simulink model "directRRR"  (R2021b)
settings: Solver=VariableStepAuto  StartTime=0.0  StopTime=10.0  RelTol=1e-3
settings Model: Creator=fabioscap  LastModifiedBy=fabioscap

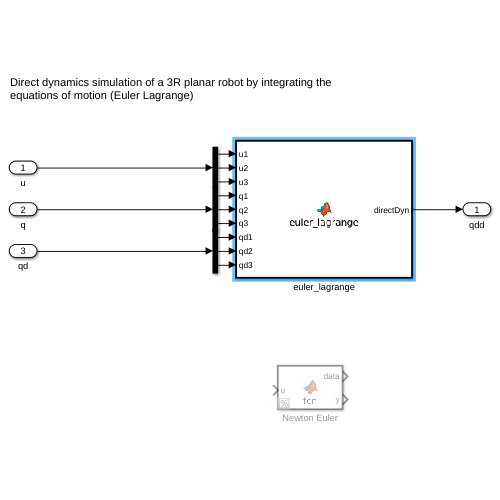
[thumbnail: Simulink's stored preview of the top-level diagram]
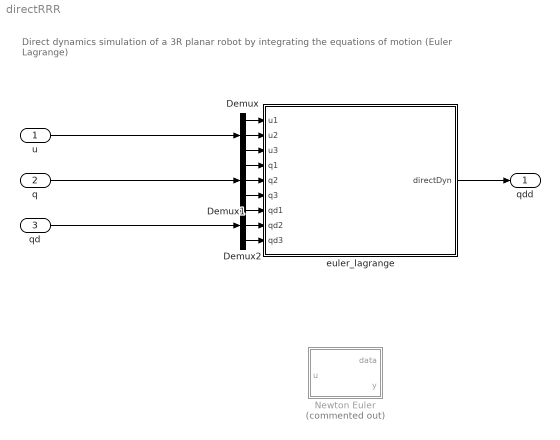
== system directRRR ==
  note: Direct dynamics simulation of a 3R planar robot by integrating the equations of motion (Euler Lagrange)
  u : Inport  PortDimensions=3
  q : Inport  Port=2  PortDimensions=3
  qd : Inport  Port=3  PortDimensions=3
  Demux : Demux  Outputs=3
  Demux1 : Demux  Outputs=3
  Demux2 : Demux  Outputs=3
  Newton Euler : MATLAB Function  Commented=on  TreatAsAtomicUnit=on
  euler_lagrange : MATLAB Function  TreatAsAtomicUnit=on
  qdd : Outport  PortDimensions=3
  wires:
  u/1 -> Demux/1
  Demux2/1 -> euler_lagrange/7(qd1)
  Demux2/3 -> euler_lagrange/9(qd3)
  Demux1/1 -> euler_lagrange/4(q1)
  Demux1/2 -> euler_lagrange/5(q2)
  Demux1/3 -> euler_lagrange/6(q3)
  Demux/3 -> euler_lagrange/3(u3)
  Demux/2 -> euler_lagrange/2(u2)
  Demux/1 -> euler_lagrange/1(u1)
  Demux2/2 -> euler_lagrange/8(qd2)
  euler_lagrange/1(directDyn) -> qdd/1
  qd/1 -> Demux2/1
  q/1 -> Demux1/1

== matlab function directRRR/euler_lagrange ==
  data: u1 input; directDyn output; u2 input; u3 input; q1 input; q2 input; q3 input; qd1 input; qd2 input; qd3 input
function directDyn = euler_lagrange(u1,u2,u3,q1,q2,q3,qd1,qd2,qd3)
%#codegen

%    This function was generated by the Symbolic Math Toolbox version 9.0.
%    20-Jul-2022 19:34:33

t2 = cos(q1);
t3 = cos(q2);
t4 = cos(q3);
t5 = sin(q1);
t6 = sin(q2);
t7 = sin(q3);
t8 = q2+q3;
t9 = qd1.^2;
t10 = qd2.^2;
t11 = qd3.^2;
t23 = u1.*5.0e+3;
t12 = t3.^2;
t13 = t3.^3;
t14 = t4.^2;
t15 = t4.^3;
t16 = t7.^2;
t17 = t7.^3;
t18 = cos(t8);
t19 = sin(t8);
t28 = t3.*u1.*2.0e+3;
t29 = t3.*u2.*2.0e+3;
t30 = t3.*u3.*2.0e+3;
t31 = t2.*1.22625e+5;
t35 = t7.*t11.*4.5e+3;
t36 = t6.*t10.*7.5e+3;
t39 = qd1.*qd3.*t7.*9.0e+3;
t40 = qd2.*qd3.*t7.*9.0e+3;
t41 = qd1.*qd2.*t6.*1.5e+4;
t46 = t3.*t4.*u3.*8.0e+2;
t48 = t2.*t3.*8.3385e+4;
t53 = t5.*t6.*1.32435e+5;
t58 = qd1.*qd2.*t3.*t7.*2.0e+3;
t59 = qd1.*qd3.*t3.*t7.*2.0e+3;
t60 = qd2.*qd3.*t3.*t7.*2.0e+3;
t61 = qd1.*qd2.*t3.*t6.*6.0e+3;
t77 = t3.*t7.*t9.*1.0e+3;
t78 = t3.*t7.*t10.*1.0e+3;
t79 = t3.*t7.*t11.*1.0e+3;
t80 = t3.*t6.*t9.*3.0e+3;
t81 = t3.*t6.*t10.*3.0e+3;
t85 = t3.*t5.*t6.*2.943e+4;
t91 = t3.*t4.*t7.*t9.*4.0e+2;
t92 = t3.*t4.*t7.*t10.*4.0e+2;
t98 = qd1.*qd2.*t3.*t4.*t7.*8.0e+2;
t128 = t2.*t4.*t6.*t7.*1.7658e+4;
t129 = t3.*t4.*t5.*t7.*1.7658e+4;
t144 = t2.*t3.*t4.*t6.*t7.*3.924e+3;
t20 = t18.^2;
t21 = t19.^2;
t22 = t19.^3;
t24 = t12.*2.0e+1;
t26 = t14.*1.44e+2;
t27 = t16.*1.8e+2;
t32 = -t29;
t33 = t14.*u1.*3.2e+3;
t34 = t14.*u2.*3.2e+3;
t37 = t16.*u1.*4.0e+3;
t38 = t16.*u2.*4.0e+3;
t42 = -t31;
t45 = t18.*u3.*2.0e+3;
t49 = -t35;
t51 = -t39;
t52 = -t40;
t55 = qd1.*qd2.*t19.*5.0e+3;
t56 = qd1.*qd3.*t19.*5.0e+3;
t57 = qd2.*qd3.*t19.*5.0e+3;
t62 = -t53;
t63 = t4.*t18.*u1.*3.2e+3;
t64 = t4.*t18.*u2.*3.2e+3;
t65 = t4.*t18.*u3.*3.2e+3;
t66 = t2.*t12.*2.943e+4;
t67 = t7.*t19.*u1.*4.0e+3;
t68 = t7.*t19.*u2.*4.0e+3;
t69 = t7.*t19.*u3.*4.0e+3;
t70 = t3.*t4.*t18.*6.4e+1;
t71 = t3.*t7.*t19.*8.0e+1;
t73 = t9.*t19.*2.5e+3;
t74 = t10.*t19.*2.5e+3;
t75 = t11.*t19.*2.5e+3;
t82 = -t58;
t83 = -t59;
t84 = -t60;
t87 = t2.*t14.*7.848e+4;
t89 = t2.*t16.*9.81e+4;
t93 = qd1.*qd2.*t3.*t19.*2.0e+3;
t94 = qd1.*qd2.*t7.*t18.*2.0e+3;
t95 = qd1.*qd3.*t3.*t19.*2.0e+3;
t96 = qd2.*qd3.*t3.*t19.*2.0e+3;
t101 = -t77;
t102 = -t78;
t103 = -t79;
t104 = -t85;
t105 = t2.*t3.*t14.*1.7658e+4;
t106 = t4.*t7.*t19.*u3.*1.6e+3;
t107 = t6.*t9.*t14.*4.8e+3;
t108 = t6.*t10.*t14.*4.8e+3;
t109 = t6.*t9.*t16.*6.0e+3;
t110 = t6.*t10.*t16.*6.0e+3;
t111 = qd1.*qd2.*t6.*t14.*9.6e+3;
t112 = t5.*t6.*t14.*1.7658e+4;
t114 = qd1.*qd2.*t6.*t16.*1.2e+4;
t118 = t3.*t9.*t19.*1.0e+3;
t119 = t7.*t9.*t18.*1.0e+3;
t120 = t3.*t10.*t19.*1.0e+3;
t121 = t7.*t10.*t18.*1.0e+3;
t122 = t3.*t11.*t19.*1.0e+3;
t123 = t4.*t9.*t19.*1.8e+3;
t124 = t16.*t18.*u3.*1.6e+3;
t125 = -t91;
t126 = -t92;
t127 = -t98;
t130 = qd1.*qd2.*t17.*t18.*1.6e+3;
t131 = qd1.*qd2.*t14.*t19.*3.2e+3;
t132 = qd1.*qd3.*t14.*t19.*3.2e+3;
t134 = qd2.*qd3.*t14.*t19.*3.2e+3;
t136 = t3.*t5.*t6.*t14.*3.924e+3;
t137 = t4.*t5.*t7.*t12.*3.924e+3;
t139 = t3.*t4.*t9.*t19.*4.0e+2;
t140 = t2.*t12.*t14.*3.924e+3;
t141 = qd1.*qd2.*t4.*t7.*t18.*3.2e+3;
t142 = qd1.*qd3.*t4.*t7.*t18.*3.2e+3;
t143 = qd2.*qd3.*t4.*t7.*t18.*3.2e+3;
t145 = t2.*t4.*t18.*7.848e+4;
t148 = t2.*t7.*t19.*9.81e+4;
t150 = t9.*t17.*t18.*8.0e+2;
t152 = t10.*t17.*t18.*8.0e+2;
t153 = t9.*t14.*t19.*1.6e+3;
t154 = t10.*t14.*t19.*1.6e+3;
t155 = t11.*t14.*t19.*1.6e+3;
t164 = t4.*t7.*t18.*t19.*1.28e+2;
t165 = t2.*t3.*t4.*t18.*5.6898e+4;
t166 = t9.*t18.*t19.*1.0e+3;
t168 = t4.*t7.*t9.*t18.*1.6e+3;
t169 = t4.*t7.*t10.*t18.*1.6e+3;
t170 = t4.*t7.*t11.*t18.*1.6e+3;
t171 = t4.*t6.*t9.*t18.*4.8e+3;
t172 = t4.*t6.*t10.*t18.*4.8e+3;
t177 = qd1.*qd2.*t4.*t6.*t18.*9.6e+3;
t178 = t2.*t6.*t7.*t18.*9.81e+3;
t179 = t3.*t5.*t7.*t18.*9.81e+3;
t180 = t4.*t5.*t6.*t18.*5.6898e+4;
t181 = t2.*t3.*t7.*t19.*5.886e+4;
t183 = t6.*t7.*t9.*t19.*6.0e+3;
t184 = t6.*t7.*t10.*t19.*6.0e+3;
t185 = qd1.*qd2.*t6.*t7.*t19.*1.2e+4;
t186 = t5.*t6.*t7.*t19.*5.886e+4;
t188 = t5.*t7.*t12.*t18.*3.924e+3;
t189 = t2.*t6.*t17.*t18.*7.848e+3;
t190 = t3.*t5.*t17.*t18.*7.848e+3;
t191 = qd1.*qd2.*t4.*t16.*t19.*1.6e+3;
t197 = t3.*t9.*t18.*t19.*4.0e+2;
t198 = qd1.*qd2.*t4.*t18.*t19.*3.2e+3;
t199 = qd1.*qd3.*t4.*t18.*t19.*3.2e+3;
t200 = qd2.*qd3.*t4.*t18.*t19.*3.2e+3;
t202 = t2.*t3.*t6.*t7.*t18.*3.924e+3;
t203 = t3.*t4.*t5.*t6.*t18.*3.924e+3;
t211 = t2.*t4.*t12.*t18.*3.924e+3;
t217 = t4.*t9.*t18.*t19.*1.6e+3;
t218 = t4.*t10.*t18.*t19.*1.6e+3;
t219 = t4.*t11.*t18.*t19.*1.6e+3;
t222 = t4.*t9.*t16.*t19.*8.0e+2;
t224 = t4.*t10.*t16.*t19.*8.0e+2;
t228 = t2.*t3.*t4.*t16.*t18.*7.848e+3;
t229 = t2.*t3.*t7.*t14.*t19.*7.848e+3;
t230 = qd1.*qd2.*t16.*t18.*t19.*1.6e+3;
t231 = t4.*t5.*t6.*t16.*t18.*7.848e+3;
t232 = t2.*t4.*t6.*t16.*t19.*7.848e+3;
t233 = t3.*t4.*t5.*t16.*t19.*7.848e+3;
t236 = t5.*t6.*t7.*t14.*t19.*7.848e+3;
t242 = t9.*t16.*t18.*t19.*8.0e+2;
t244 = t10.*t16.*t18.*t19.*8.0e+2;
t247 = t2.*t3.*t4.*t7.*t18.*t19.*7.848e+3;
t248 = t4.*t5.*t6.*t7.*t18.*t19.*7.848e+3;
t249 = t2.*t6.*t16.*t18.*t19.*7.848e+3;
t250 = t3.*t5.*t16.*t18.*t19.*7.848e+3;
t25 = -t24;
t43 = t20.*8.0e+1;
t44 = t21.*1.0e+2;
t47 = -t34;
t50 = -t38;
t54 = -t45;
t72 = t20.*u2.*3.2e+3;
t76 = t21.*u2.*4.0e+3;
t86 = -t64;
t88 = -t68;
t90 = -t70;
t97 = -t71;
t113 = -t87;
t115 = -t89;
t116 = t16.*t20.*6.4e+1;
t117 = t14.*t21.*6.4e+1;
t133 = qd1.*qd3.*t7.*t20.*3.2e+3;
t135 = qd2.*qd3.*t7.*t20.*3.2e+3;
t138 = -t105;
t146 = -t123;
t147 = -t124;
t149 = t2.*t3.*t20.*4.7088e+4;
t151 = t4.*t9.*t22.*8.0e+2;
t156 = t7.*t11.*t20.*1.6e+3;
t157 = t6.*t9.*t20.*4.8e+3;
t158 = t2.*t3.*t21.*5.886e+4;
t159 = t6.*t9.*t21.*6.0e+3;
t162 = t5.*t6.*t20.*4.7088e+4;
t163 = t5.*t6.*t21.*5.886e+4;
t167 = -t139;
t173 = -t140;
t174 = -t141;
t175 = -t142;
t176 = -t143;
t182 = -t145;
t187 = -t148;
t192 = qd1.*qd2.*t4.*t7.*t21.*1.6e+3;
t201 = -t164;
t204 = -t168;
t205 = -t169;
t206 = -t170;
t207 = -t178;
t208 = -t179;
t209 = -t180;
t210 = -t186;
t212 = -t188;
t213 = -t189;
t214 = -t190;
t215 = -t191;
t220 = -t202;
t221 = -t203;
t223 = t4.*t7.*t9.*t21.*8.0e+2;
t225 = t4.*t7.*t10.*t21.*8.0e+2;
t226 = t2.*t3.*t14.*t21.*7.848e+3;
t227 = t5.*t6.*t14.*t21.*7.848e+3;
t234 = t2.*t4.*t6.*t7.*t21.*7.848e+3;
t235 = t3.*t4.*t5.*t7.*t21.*7.848e+3;
t237 = -t222;
t239 = -t224;
t243 = t7.*t9.*t18.*t21.*8.0e+2;
t245 = -t229;
t246 = -t231;
t251 = -t248;
t252 = -t249;
t253 = -t250;
t99 = -t72;
t100 = -t76;
t160 = -t133;
t161 = -t135;
t193 = -t151;
t194 = -t156;
t195 = -t162;
t196 = -t163;
t216 = -t192;
t238 = -t223;
t240 = -t225;
t241 = -t226;
t254 = t25+t26+t27+t43+t44+t90+t97+t116+t117+t201+2.25e+2;
t255 = 1.0./t254;
et1 = t23+t28+t30+t33+t36+t37+t41+t42+t46+t47+t48+t49+t50+t51+t52+t54+t55+t56+t57+t61+t62+t63+t65+t66+t67+t69+t73+t74+t75+t81+t82+t83+t84+t93+t94+t95+t96+t99+t100+t101+t102+t103+t104+t106+t107+t108+t109+t110+t111+t112+t113+t114+t115+t118+t119+t120+t121+t122+t125+t126+t127+t128+t129+t130+t131+t132+t134+t136+t137+t138+t144+t146+t147+t149+t150+t152+t153+t154+t155+t157+t158+t159+t160+t161+t165+t166+t167+t172+t173+t174+t175+t176+t177+t181+t182+t184+t185+t187+t193+t194+t195+t196+t197+t198+t199+t200+t204+t205+t206+t207+t208+t209+t210+t211+t212+t213+t214+t215+t216+t217+t218+t219+t220+t221+t227+t228+t230+t232+t233+t234+t235+t236+t237+t239+t240+t241+t243+t244+t245+t246+t247+t251+t252+t253-u2.*1.4e+4+u3.*9.0e+3+t6.*t9.*2.1e+4-t7.*t9.*4.5e+3-t7.*t10.*4.5e+3-t3.*u2.*4.0e+3+t4.*u3.*3.6e+3;
et2 = t20.*u3.*3.2e+3+t21.*u3.*4.0e+3-qd1.*qd2.*t7.*9.0e+3+t3.*t6.*t9.*6.0e+3-t4.*t7.*t9.*1.8e+3-t4.*t7.*t10.*1.8e+3-t7.*t9.*t20.*1.6e+3-t7.*t10.*t20.*1.6e+3-t3.*t18.*u3.*8.0e+2-t4.*t18.*u2.*6.4e+3+t4.*t21.*u3.*1.6e+3-t7.*t19.*u2.*8.0e+3-qd1.*qd2.*t4.*t7.*3.6e+3-qd1.*qd2.*t7.*t20.*3.2e+3+t3.*t7.*t9.*t18.*4.0e+2+t4.*t6.*t9.*t18.*9.6e+3+t3.*t7.*t10.*t18.*4.0e+2-t4.*t7.*t9.*t21.*1.6e+3+t6.*t7.*t9.*t19.*1.2e+4+t9.*t16.*t18.*t19.*1.6e+3-t7.*t18.*t19.*u3.*1.6e+3+qd1.*qd2.*t3.*t7.*t18.*8.0e+2;
et3 = t28+t32+t48+t49+t51+t52+t61+t62+t63+t67+t80+t81+t86+t88+t93+t95+t96+t99+t100+t112+t118+t120+t122+t128+t129+t138+t139+t146+t149+t157+t158+t159+t160+t161-t166+t171+t172+t177+t182+t183+t184+t185+t187+t193+t194+t195+t196+t197+t198+t199+t200+t211+t212+t216+t217+t218+t219+t220+t221+t227+t230+t234+t235+t238+t240+t241+t242+t243+t244+t247+t251+t252+t253-u2.*9.0e+3+u3.*1.8e+4+t6.*t9.*1.35e+4-t7.*t9.*9.0e+3-t7.*t10.*9.0e+3+t2.*t18.*4.905e+4-t9.*t17.*3.6e+3-t10.*t17.*3.6e+3-t9.*t19.*4.5e+3-t9.*t22.*2.0e+3+t3.*t141+t3.*t168+t3.*t169+t3.*t217-t4.*u2.*3.6e+3+t4.*u3.*7.2e+3-t12.*u3.*8.0e+2+t14.*u3.*7.2e+3;
et4 = t16.*u3.*7.2e+3-t18.*u1.*2.0e+3+t18.*u2.*2.0e+3+t20.*u3.*7.2e+3+t21.*u3.*8.0e+3-qd1.*qd2.*t7.*1.8e+4-qd1.*qd2.*t17.*7.2e+3-t2.*t3.*t4.*1.0791e+4+t2.*t6.*t7.*4.4145e+4+t3.*t5.*t7.*4.4145e+4-t4.*t5.*t6.*8.829e+3+t2.*t4.*t13.*3.924e+3+t4.*t6.*t9.*5.4e+3-t2.*t3.*t15.*3.5316e+4-t4.*t7.*t9.*3.6e+3-t4.*t7.*t10.*3.6e+3-t4.*t7.*t11.*1.8e+3+t2.*t6.*t17.*3.5316e+4+t3.*t5.*t17.*3.5316e+4-t5.*t7.*t13.*3.924e+3+t5.*t6.*t15.*3.5316e+4+t7.*t9.*t12.*4.0e+2+t7.*t10.*t12.*4.0e+2;
et5 = t7.*t9.*t14.*-3.6e+3-t7.*t10.*t14.*3.6e+3-t2.*t12.*t18.*1.1772e+4-t6.*t9.*t18.*3.0e+3-t6.*t10.*t18.*3.0e+3+t2.*t16.*t18.*3.924e+4-t7.*t9.*t20.*3.6e+3-t7.*t9.*t21.*2.0e+3-t7.*t10.*t20.*3.6e+3-t7.*t10.*t21.*2.0e+3+t9.*t12.*t19.*4.0e+2-t9.*t14.*t19.*3.6e+3-t9.*t16.*t19.*3.6e+3-t9.*t14.*t22.*1.6e+3-t9.*t17.*t20.*1.6e+3-t10.*t17.*t20.*1.6e+3-t10.*t18.*t19.*1.0e+3-t9.*t19.*t20.*2.0e+3-t11.*t18.*t19.*1.0e+3+t3.*t4.*u1.*8.0e+2-t3.*t4.*u2.*8.0e+2+t3.*t18.*u2.*8.0e+2;
et6 = t3.*t18.*u3.*-1.6e+3-t4.*t21.*u2.*1.6e+3+t4.*t21.*u3.*3.2e+3-t16.*t18.*u1.*1.6e+3+t16.*t18.*u2.*1.6e+3+t14.*t21.*u3.*3.2e+3+t16.*t20.*u3.*3.2e+3-qd1.*qd2.*t4.*t7.*7.2e+3-qd1.*qd3.*t4.*t7.*3.6e+3-qd2.*qd3.*t4.*t7.*3.6e+3+qd1.*qd2.*t7.*t12.*8.0e+2-qd1.*qd2.*t7.*t14.*7.2e+3-qd1.*qd2.*t6.*t18.*6.0e+3-qd1.*qd2.*t7.*t20.*7.2e+3-qd1.*qd2.*t7.*t21.*4.0e+3-qd1.*qd2.*t17.*t20.*3.2e+3-qd1.*qd2.*t18.*t19.*2.0e+3-qd1.*qd3.*t18.*t19.*2.0e+3-qd2.*qd3.*t18.*t19.*2.0e+3+t3.*t4.*t6.*t9.*1.2e+3+t3.*t4.*t6.*t10.*1.2e+3;
et7 = t2.*t3.*t4.*t16.*-3.5316e+4-t2.*t6.*t7.*t12.*3.924e+3-t4.*t5.*t6.*t12.*3.924e+3-t2.*t3.*t4.*t20.*1.962e+4+t2.*t6.*t7.*t14.*3.5316e+4+t3.*t5.*t7.*t14.*3.5316e+4+t2.*t3.*t4.*t21.*3.924e+3+t4.*t5.*t6.*t16.*3.5316e+4-t2.*t4.*t7.*t19.*3.924e+4+t3.*t5.*t6.*t18.*1.1772e+4+t2.*t6.*t7.*t20.*1.962e+4+t3.*t5.*t7.*t20.*1.962e+4+t4.*t5.*t6.*t20.*1.962e+4+t2.*t6.*t7.*t21.*1.962e+4+t3.*t4.*t10.*t19.*4.0e+2+t3.*t5.*t7.*t21.*1.962e+4-t3.*t6.*t9.*t18.*1.2e+3-t4.*t5.*t6.*t21.*3.924e+3+t3.*t4.*t11.*t19.*4.0e+2+t3.*t7.*t9.*t18.*8.0e+2;
et8 = t3.*t7.*t10.*t18.*8.0e+2+t3.*t7.*t11.*t18.*4.0e+2+t3.*t7.*t9.*t21.*1.6e+3+t4.*t6.*t9.*t21.*2.4e+3-t2.*t3.*t15.*t21.*1.5696e+4+t2.*t6.*t17.*t20.*1.5696e+4+t3.*t5.*t17.*t20.*1.5696e+4+t2.*t12.*t14.*t18.*1.5696e+4+t3.*t9.*t16.*t19.*1.6e+3+t5.*t6.*t15.*t21.*1.5696e+4+t3.*t10.*t16.*t19.*1.6e+3-t6.*t9.*t16.*t18.*2.4e+3-t6.*t10.*t16.*t18.*2.4e+3-t7.*t9.*t14.*t21.*1.6e+3-t5.*t12.*t16.*t19.*1.5696e+4-t7.*t10.*t14.*t21.*1.6e+3-t9.*t16.*t19.*t20.*1.6e+3-t3.*t4.*t18.*u3.*3.2e+3+t4.*t7.*t19.*u1.*1.6e+3-t3.*t7.*t19.*u3.*3.2e+3;
et9 = t4.*t7.*t19.*u2.*-1.6e+3+t7.*t18.*t19.*u2.*1.6e+3-t7.*t18.*t19.*u3.*3.2e+3+qd1.*qd2.*t3.*t4.*t6.*2.4e+3+qd1.*qd2.*t3.*t4.*t19.*8.0e+2+qd1.*qd3.*t3.*t4.*t19.*8.0e+2+qd1.*qd2.*t3.*t7.*t18.*1.6e+3+qd2.*qd3.*t3.*t4.*t19.*8.0e+2+qd1.*qd3.*t3.*t7.*t18.*8.0e+2+qd2.*qd3.*t3.*t7.*t18.*8.0e+2+qd1.*qd2.*t3.*t16.*t19.*3.2e+3-qd1.*qd2.*t6.*t16.*t18.*4.8e+3-qd1.*qd2.*t7.*t14.*t21.*3.2e+3+t2.*t4.*t7.*t12.*t19.*1.5696e+4-t2.*t3.*t4.*t16.*t20.*1.5696e+4+t4.*t6.*t7.*t9.*t19.*2.4e+3-t2.*t3.*t6.*t16.*t19.*1.5696e+4-t3.*t5.*t6.*t14.*t18.*1.5696e+4-t4.*t5.*t7.*t12.*t18.*1.5696e+4;
et10 = t4.*t6.*t7.*t10.*t19.*2.4e+3-t2.*t3.*t7.*t18.*t19.*2.3544e+4+t2.*t6.*t7.*t14.*t21.*1.5696e+4+t3.*t5.*t7.*t14.*t21.*1.5696e+4+t4.*t5.*t6.*t16.*t20.*1.5696e+4+t5.*t6.*t7.*t18.*t19.*2.3544e+4+t4.*t7.*t9.*t18.*t21.*3.2e+3-t6.*t7.*t9.*t18.*t19.*2.4e+3+t4.*t9.*t16.*t18.*t19.*3.2e+3+t4.*t10.*t16.*t18.*t19.*3.2e+3-t4.*t7.*t18.*t19.*u3.*6.4e+3+qd1.*qd2.*t4.*t6.*t7.*t19.*4.8e+3+qd1.*qd2.*t4.*t16.*t18.*t19.*6.4e+3-t2.*t3.*t4.*t6.*t7.*t18.*1.5696e+4-t3.*t4.*t5.*t6.*t7.*t19.*1.5696e+4+t2.*t3.*t7.*t14.*t18.*t19.*3.1392e+4-t2.*t4.*t6.*t16.*t18.*t19.*3.1392e+4;
et11 = t3.*t4.*t5.*t16.*t18.*t19.*-3.1392e+4-t5.*t6.*t7.*t14.*t18.*t19.*3.1392e+4;
directDyn = [(t255.*(t23+t30+t32+t33+t36+t37+t41+t42+t46+t47+t50+t54+t55+t56+t57+t65+t66+t69+t73+t74+t75+t80+t82+t83+t84+t86+t88+t94+t101+t102+t103+t104+t106+t107+t108+t109+t110+t111+t113+t114+t115+t119+t121+t125+t126+t127+t130+t131+t132+t134+t136+t137+t144+t147+t150+t152+t153+t154+t155+t165+t166+t167+t171+t173+t174+t175+t176+t181+t183+t204+t205+t206+t207+t208+t209+t210+t213+t214+t215+t228+t232+t233+t236+t237+t238+t239+t242+t245+t246-u2.*5.0e+3+t6.*t9.*7.5e+3))./5.0e+1;t255.*(et1+et2).*(-1.0./5.0e+1);(t255.*(et3+et4+et5+et6+et7+et8+et9+et10+et11))./5.0e+1];

== matlab function directRRR/Newton Euler ==
  data: data output; u input; y output
function [data, y]= fcn(u)

y = u;
